simulink model "Kal_noPitch_sim"  (R2023b)
settings: Solver=FixedStepAuto  StartTime=0.0  StopTime=50  FixedStep=0.001  RelTol=1e-3
values from neighbouring files (symbols this model uses):
  beta = pi/10    (= 0.314159265359)    [Kal_noPitch_mat.m]
  cov_ic = cov_ic * (1 + 2*rand)    [Kal_noPitch_mat.m]
  des_vel = [0.1, 0, 0, 0]'    [Kal_noPitch_mat.m]
  eta1 = 0.05    [Kal_noPitch_mat.m]
  eta2 = 0.05    [Kal_noPitch_mat.m]
  G = eye(3) * Ts    [Kal_noPitch_mat.m]
  Gamma = -pi/6    (= -0.523598775598)    [Kal_noPitch_mat.m]
  h_ref = 7    [Kal_noPitch_mat.m]
  init_cond = [2; 0; 0]    [Kal_noPitch_mat.m]
  Kd_dep = (p + 2*damp*wn)*mv(3) + dv(3)    [Control_gains_mat.m]
  Ki_dep = p*(wn^2)*mv(3)    [Control_gains_mat.m]
  Ki_surge = wn^2 * mv(1)    [Control_gains_mat.m]
  Kp_dep = mv(3)*((wn^2) + 2*damp*p*wn)    [Control_gains_mat.m]
  Kp_surge = 2*damp*wn*mv(1) - dv(1)    [Control_gains_mat.m]
  Kt_dep = 1 / sqrt(ti_dep*td_dep)    [Control_gains_mat.m]
  Kt_surge = 1 / ti_surge    [Control_gains_mat.m]
  Lambda = pi/6    (= 0.523598775598)    [Kal_noPitch_mat.m]
  pr0 = [0,0]'    [Kal_noPitch_mat.m]
  Q = zeros(3,3)    [Kal_noPitch_mat.m]
  qt = - 10    (= -10)    [Kal_noPitch_mat.m]
  R = [(eta1^2), 0 ... (first row only)    [Kal_noPitch_mat.m]
  sat_dep = 15    [Model3D_equation_mat.m]
  sat_surge = 15    [Model3D_equation_mat.m]
  sat_tr = 2000    [Model3D_equation_mat.m]
  sig1 = 0.1    [Kal_noPitch_mat.m]
  sig2 = 0.2    [Kal_noPitch_mat.m]
  sig3 = 0.15    [Kal_noPitch_mat.m]
  speed0 = [0.1, 0, 0, 0]'    [Model3D_equation_mat.m]
  Ts = 0.001    [Kal_noPitch_mat.m]
settings Model: Creator=fabio  LastModifiedBy=fabio

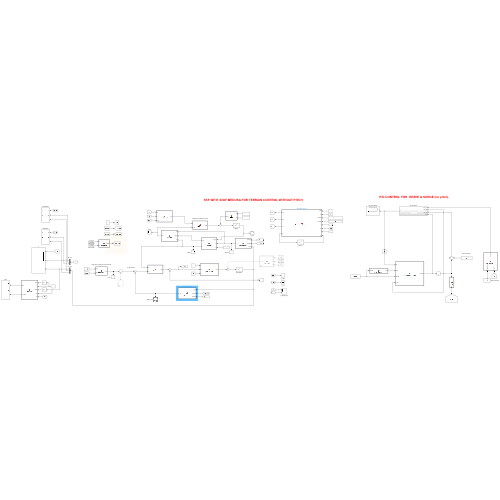
[thumbnail: Simulink's stored preview of the top-level diagram]
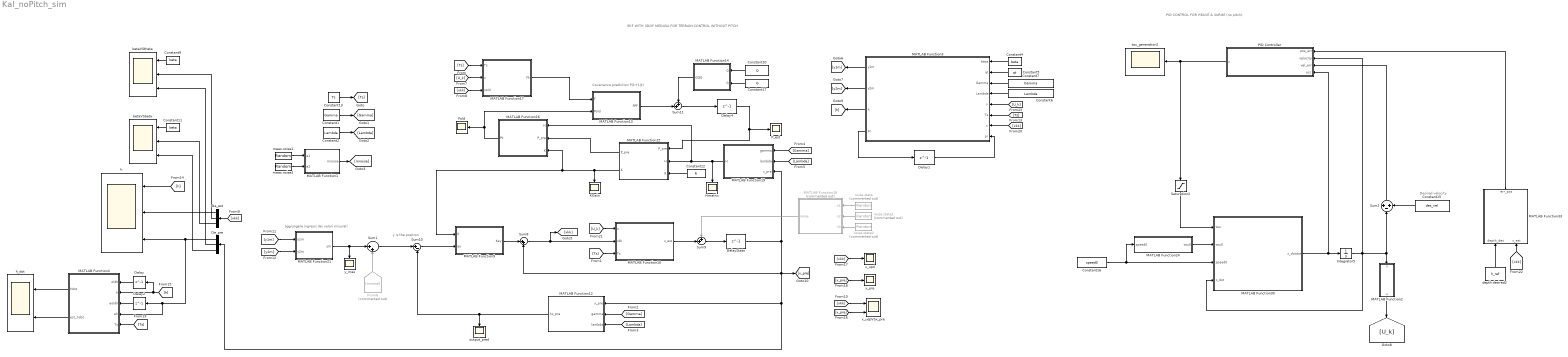
== system Kal_noPitch_sim ==
  note: aggiungere ingressi dei valorì misurati
  note: Covariance prediction P(k+1|k)
  note: EKF WITH 3DOF MEDUSA FOR TERRAIN CONTROL WITHOUT PITCH
  note: y is the position
  note: PID CONTROL FOR HEAVE & SURGE (no pitch).
  note: Desired velocity
  Constant1 : Constant  Value=Gamma
  Constant10 : Constant  Value=Q  VectorParams1D=off
  Constant11 : Constant  Value=beta
  Constant12 : Constant  Value=R
  Constant13 : Constant  Value=Ts
  Constant15 : Constant  Value=des_vel
  Constant16 : Constant  Value=speed0
  Constant17 : Constant  Value=G  VectorParams1D=off
  Constant2 : Constant  Value=Lambda
  Constant4 : Constant  Value=beta
  Constant5 : Constant  Value=qt
  Constant6 : Constant  Value=Lambda
  Constant7 : Constant  Value=Gamma
  Constant9 : Constant  Value=beta
  De_est : Demux  Outputs=3
  De_pre : Demux  Outputs=3
  Delay : Delay  DelayLength=1
  Delay1 : Delay  DelayLength=1  InitialCondition=pr0  UseCircularBuffer=on
  Delay2 : Delay  DelayLength=1
  Delay4 : Delay  DelayLength=1  InitialCondition=cov_ic  UseCircularBuffer=on
  DelayStato : Delay  DelayLength=1  InitialCondition=init_cond  UseCircularBuffer=on
  From6 : From  Commented=on  GotoTag=mnoise
  Hmatrix : Scope
  Integrator5 : Integrator
  KGain : Scope
  MATLAB Function1 : MATLAB Function  TreatAsAtomicUnit=on
  MATLAB Function10 : MATLAB Function  TreatAsAtomicUnit=on
  MATLAB Function12 : MATLAB Function  TreatAsAtomicUnit=on
  MATLAB Function13 : MATLAB Function  TreatAsAtomicUnit=on
  MATLAB Function14 : MATLAB Function  TreatAsAtomicUnit=on
  MATLAB Function15 : MATLAB Function  TreatAsAtomicUnit=on
  MATLAB Function16 : MATLAB Function  TreatAsAtomicUnit=on
  MATLAB Function17 : MATLAB Function  TreatAsAtomicUnit=on
  MATLAB Function18 : MATLAB Function  Commented=on  TreatAsAtomicUnit=on
  MATLAB Function19 : MATLAB Function  TreatAsAtomicUnit=on
  MATLAB Function2 : MATLAB Function  TreatAsAtomicUnit=on
  MATLAB Function21 : MATLAB Function  TreatAsAtomicUnit=on
  MATLAB Function24 : MATLAB Function  TreatAsAtomicUnit=on
  MATLAB Function3 : MATLAB Function  TreatAsAtomicUnit=on
  MATLAB Function30 : MATLAB Function  TreatAsAtomicUnit=on
  MATLAB Function33 : MATLAB Function  TreatAsAtomicUnit=on
  MATLAB Function4 : MATLAB Function  TreatAsAtomicUnit=on
  MATLAB Function9 : MATLAB Function  TreatAsAtomicUnit=on
  PID Controller : Subsystem
  P_est : Scope
  Pold : Scope
  Saturation2 : Saturate  UpperLimit=sat_tr  LowerLimit=-sat_tr
  Sum1 : Sum  Inputs=|++
  Sum10 : Sum  Inputs=|+-
  Sum11 : Sum  Inputs=++|
  Sum2 : Sum  Inputs=+-+
  Sum8 : Sum  Inputs=|++
  Sum9 : Sum  Inputs=++|
  betaVSbeta : Scope  NumInputPorts=3
  betaVStheta : Scope  NumInputPorts=3
  depth desired2 : Constant  Value=h_ref
  h : Scope  NumInputPorts=3
  h_dot : Scope  NumInputPorts=2
  meas.noise1 : RandomNumber  Variance=eta1  SampleTime=Ts
  meas.noise2 : RandomNumber  Variance=eta2  SampleTime=Ts
  noise state : RandomNumber  Commented=on  Variance=sig1  SampleTime=Ts
  noise state1 : RandomNumber  Commented=on  Variance=sig2  SampleTime=Ts
  noise state2 : RandomNumber  Commented=on  Variance=sig3  SampleTime=Ts
  output_pred : Scope
  tau_generation2 : Scope
  x_pre : Scope
  x_udpVSx_pre : Scope  NumInputPorts=2
  x_upd : Scope
  y_mes : Scope
  wires:
  MATLAB Function17/1(Fk) -> MATLAB Function13/1(F)
  DelayStato/1 -> Sum8/2, [x_pre], MATLAB Function12/1(x_pre), De_pre/1, MATLAB Function19/3(x_pre)
  Delay4/1 -> P_est/1, MATLAB Function15/1("P_pre ")
  MATLAB Function12/1(hx_pre) -> Sum10/2, output_pred/1
  Sum10/1 -> MATLAB Function9/2(ey)
  MATLAB Function19/1(H) -> Hmatrix/1, MATLAB Function16/1(H), MATLAB Function15/2(H)
  Constant17/1 -> MATLAB Function14/2(G)
  MATLAB Function14/1(GQG) -> Sum11/1
  MATLAB Function13/1(FPF) -> Sum11/2
  Constant10/1 -> MATLAB Function14/1(Q)
  MATLAB Function10/1(x_est) -> Sum9/2
  MATLAB Function16/1(Pk) -> Pold/1, MATLAB Function13/2(Pold)
  Sum9/1 -> DelayStato/1
  Constant12/1 -> MATLAB Function15/3(R)
  MATLAB Function15/2(K) -> KGain/1, MATLAB Function16/3(K), MATLAB Function9/1(K)
  Sum11/1 -> Delay4/1
  Sum8/1 -> [xkk], MATLAB Function10/2(xkk)
  MATLAB Function15/1(P_pre) -> MATLAB Function16/2(P_pre)
  MATLAB Function9/1(Key) -> Sum8/1
  MATLAB Function21/1(ym) -> y_mes/1, Sum1/1
  Constant13/1 -> [Ts]
  [Ts] -> MATLAB Function17/1(Ts)
  [Ts] -> MATLAB Function10/3(Ts)
  Constant1/1 -> [Gamma]
  Constant2/1 -> [Lambda]
  [Gamma] -> MATLAB Function12/2(gamma)
  [Lambda] -> MATLAB Function12/3(lambda)
  [Gamma] -> MATLAB Function19/1(gamma)
  [Lambda] -> MATLAB Function19/2(lambda)
  noise state/1 -> MATLAB Function18/1(n1)
  noise state2/1 -> MATLAB Function18/3(n3)
  noise state1/1 -> MATLAB Function18/2(n2)
  MATLAB Function18/1(noise) -> Sum9/1
  Sum1/1 -> Sum10/1
  meas.noise1/1 -> MATLAB Function1/1(e1)
  meas.noise2/1 -> MATLAB Function1/2(e2)
  MATLAB Function1/1(mnoise) -> [mnoise]
  [U_k] -> MATLAB Function17/2(u)
  [xkk] -> MATLAB Function17/3(xold)
  Delay1/1 -> MATLAB Function3/8("pr ")
  MATLAB Function3/4(pr) -> Delay1/1
  MATLAB Function3/1(y1m) -> [y1m]
  MATLAB Function3/2(y2m) -> [y2m]
  [y1m] -> MATLAB Function21/1(y1m)
  [y2m] -> MATLAB Function21/2(y2m)
  Constant4/1 -> MATLAB Function3/1(beta)
  Constant5/1 -> MATLAB Function3/2(qt)
  Constant6/1 -> MATLAB Function3/4(Lambda)
  [U_k] -> MATLAB Function3/5(v)
  [Ts] -> MATLAB Function3/6(Ts)
  MATLAB Function3/3(h) -> [h]
  [h] -> h/1
  [xkk] -> De_est/1
  De_est/1 -> h/2
  De_pre/1 -> MATLAB Function4/4(eh), Delay2/1, h/3
  Constant9/1 -> betaVStheta/1
  Constant7/1 -> MATLAB Function3/3(Gamma)
  MATLAB Function4/1(hdot) -> h_dot/1
  De_est/2 -> betaVStheta/2
  De_pre/2 -> betaVStheta/3
  De_est/3 -> betaVSbeta/2
  De_pre/3 -> betaVSbeta/3
  Constant11/1 -> betaVSbeta/1
  [xkk] -> x_udpVSx_pre/1
  [x_pre] -> x_udpVSx_pre/2
  [xkk] -> x_upd/1
  [x_pre] -> x_pre/1
  MATLAB Function4/2(est_hdot) -> h_dot/2
  [h] -> Delay/1, MATLAB Function4/2(h)
  Delay/1 -> MATLAB Function4/1(oldh)
  Delay2/1 -> MATLAB Function4/3(eoldh)
  [Ts] -> MATLAB Function4/5(Ts)
  [xkk] -> MATLAB Function3/7(x)
  From6/1 -> Sum1/2
  Integrator5/1 -> PID Controller/2(velocity), MATLAB Function30/4(x_dot), Sum2/2, MATLAB Function2/1(x)
  MATLAB Function24/1(tau0) -> MATLAB Function30/2(tau0)
  Constant16/1 -> MATLAB Function30/3(speed0), MATLAB Function24/1(speed0)
  Sum2/1 -> PID Controller/3(vel_err)
  PID Controller/1(u) -> tau_generation2/1, Saturation2/1
  MATLAB Function33/1(err_pos) -> PID Controller/1(pos_err)
  MATLAB Function30/1(x_dotdot) -> Integrator5/1, PID Controller/4(acc)
  Saturation2/1 -> MATLAB Function30/1(tau)
  depth desired2/1 -> MATLAB Function33/1(depth_des)
  Constant15/1 -> Sum2/3
  [U_k] -> MATLAB Function10/1(u)
  MATLAB Function2/1(u) -> [U_k]
  [xkk] -> MATLAB Function33/2(x_est)

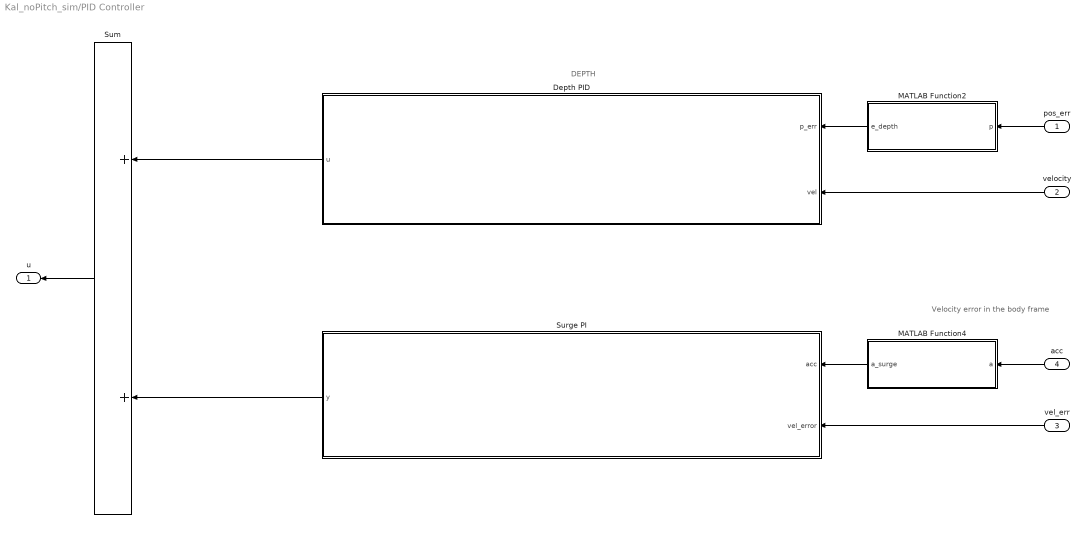
== system Kal_noPitch_sim/PID Controller ==
  note: Velocity error in the body frame
  note: DEPTH
  pos_err : Inport
  velocity : Inport  Port=2
  vel_err : Inport  Port=3
  acc : Inport  Port=4
  Depth PID : Subsystem
  MATLAB Function2 : MATLAB Function  TreatAsAtomicUnit=on
  MATLAB Function4 : MATLAB Function  TreatAsAtomicUnit=on
  Sum : Sum
  Surge PI : Subsystem
  u : Outport
  wires:
  velocity/1 -> Depth PID/2(vel)
  vel_err/1 -> Surge PI/2(vel_error)
  MATLAB Function4/1(a_surge) -> Surge PI/1(acc)
  acc/1 -> MATLAB Function4/1(a)
  Surge PI/1(y) -> Sum/2
  Sum/1 -> u/1
  Depth PID/1(u) -> Sum/1
  pos_err/1 -> MATLAB Function2/1(p)
  MATLAB Function2/1(e_depth) -> Depth PID/1(p_err)

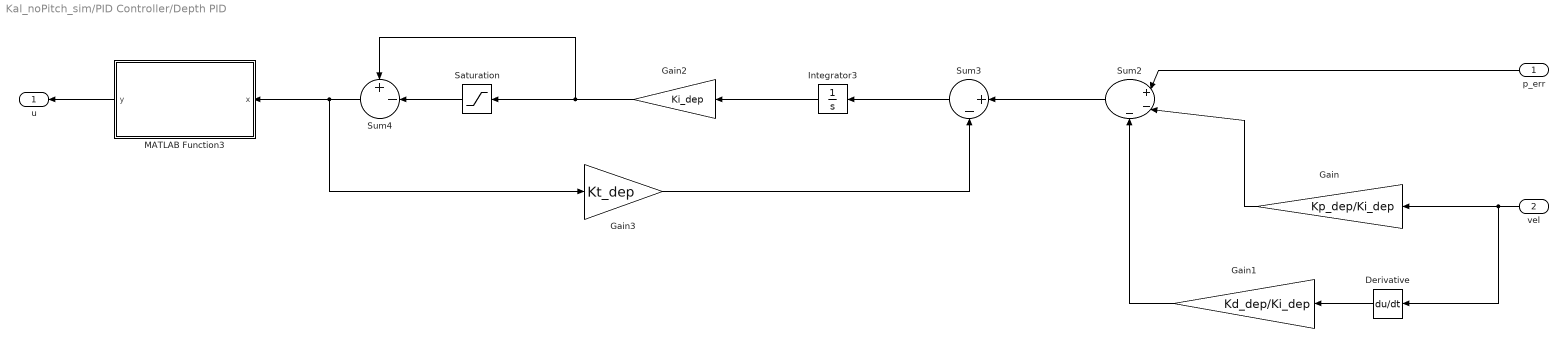
== system Kal_noPitch_sim/PID Controller/Depth PID ==
  p_err : Inport
  vel : Inport  Port=2
  Derivative : Derivative
  Gain : Gain  Gain=Kp_dep/Ki_dep
  Gain1 : Gain  Gain=Kd_dep/Ki_dep
  Gain2 : Gain  Gain=Ki_dep
  Gain3 : Gain  Gain=Kt_dep
  Integrator3 : Integrator
  MATLAB Function3 : MATLAB Function  TreatAsAtomicUnit=on
  Saturation : Saturate  UpperLimit=sat_dep  LowerLimit=-sat_dep
  Sum2 : Sum  Inputs=|+--
  Sum3 : Sum  Inputs=|+-
  Sum4 : Sum  Inputs=+-|
  u : Outport
  wires:
  Sum3/1 -> Integrator3/1
  Integrator3/1 -> Gain2/1
  Gain2/1 -> Sum4/1, Saturation/1
  Sum4/1 -> MATLAB Function3/1(x), Gain3/1
  Derivative/1 -> Gain1/1
  Saturation/1 -> Sum4/2
  Sum2/1 -> Sum3/1
  Gain/1 -> Sum2/2
  Gain1/1 -> Sum2/3
  p_err/1 -> Sum2/1
  vel/1 -> Derivative/1, Gain/1
  MATLAB Function3/1(y) -> u/1
  Gain3/1 -> Sum3/2

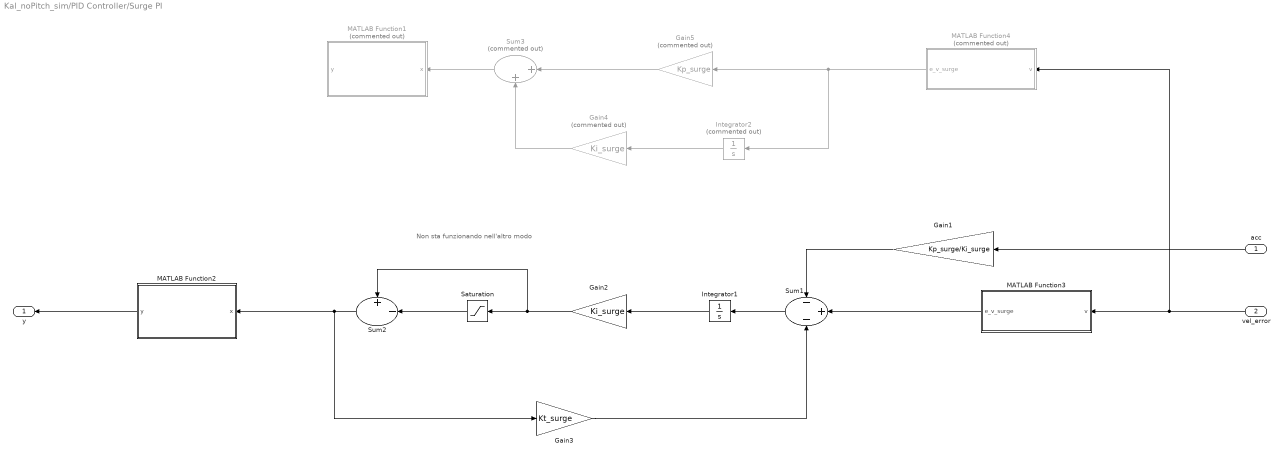
== system Kal_noPitch_sim/PID Controller/Surge PI ==
  note: Non sta funzionando nell'altro modo
  acc : Inport
  vel_error : Inport  Port=2
  Gain1 : Gain  Gain=Kp_surge/Ki_surge
  Gain2 : Gain  Gain=Ki_surge
  Gain3 : Gain  Gain=Kt_surge
  Gain4 : Gain  Commented=on  Gain=Ki_surge
  Gain5 : Gain  Commented=on  Gain=Kp_surge
  Integrator1 : Integrator
  Integrator2 : Integrator  Commented=on
  MATLAB Function1 : MATLAB Function  Commented=on  TreatAsAtomicUnit=on
  MATLAB Function2 : MATLAB Function  TreatAsAtomicUnit=on
  MATLAB Function3 : MATLAB Function  TreatAsAtomicUnit=on
  MATLAB Function4 : MATLAB Function  Commented=on  TreatAsAtomicUnit=on
  Saturation : Saturate  UpperLimit=sat_surge  LowerLimit=-sat_surge
  Sum1 : Sum  Inputs=-+-
  Sum2 : Sum  Inputs=+-|
  Sum3 : Sum  Commented=on  Inputs=|++
  y : Outport
  wires:
  Gain1/1 -> Sum1/1
  Sum2/1 -> Gain3/1, MATLAB Function2/1(x)
  Sum1/1 -> Integrator1/1
  Gain3/1 -> Sum1/3
  Saturation/1 -> Sum2/2
  Gain2/1 -> Sum2/1, Saturation/1
  Integrator1/1 -> Gain2/1
  MATLAB Function3/1(e_v_surge) -> Sum1/2
  Integrator2/1 -> Gain4/1
  vel_error/1 -> MATLAB Function3/1(v), MATLAB Function4/1(v)
  Gain5/1 -> Sum3/1
  Gain4/1 -> Sum3/2
  Sum3/1 -> MATLAB Function1/1(x)
  MATLAB Function4/1(e_v_surge) -> Integrator2/1, Gain5/1
  acc/1 -> Gain1/1
  MATLAB Function2/1(y) -> y/1

== matlab function Kal_noPitch_sim/MATLAB Function14 ==
  data: Q input; GQG output; G input
function GQG = GmatrixQ(Q, G)
    GQG = G*Q*(G');

== matlab function Kal_noPitch_sim/MATLAB Function15 ==
  data: P_pre output; P_pre input; H input; K output; R input
function [P_pre, K] = KalmanGain(P_pre, H, R)
    K = (P_pre*(H'))*pinv((H*P_pre*(H') + R)); 
    K(2,:) = 0; % non sto ancora curando theta

== matlab function Kal_noPitch_sim/MATLAB Function16 ==
  data: H input; P_pre input; Pk output; K input
function Pk = PkComp(H ,P_pre, K)
    s = size((K*H), 1);
    I = eye(s); 
    Pk = (I - K*H)*P_pre;

== matlab function Kal_noPitch_sim/MATLAB Function9 ==
  data: K input; ey input; Key output
function Key = GainMult(K, ey)
    Key = K*ey;

== matlab function Kal_noPitch_sim/MATLAB Function17 ==
  data: Fk output; Ts input; u input; xold input
function Fk = DynamicJacobian(Ts, u, xold)
    delta = xold(3) - xold(2);
    % u(1) = vsurge, u(2) = vheave
    % !! ATTENZIONE:
    % STO CONSIDERANDO H RISPETTO TERRAIN FRAME E THETA E BETA RISPETTO
    % INERZIALE
    F = [0, -u(1)*cos(delta)+u(2)*sin(delta), u(1)*cos(delta)-u(2)*sin(delta);
            0, 0, 0;
            0, 0, 0];
    Fk = eye(3) + Ts * F;

== matlab function Kal_noPitch_sim/MATLAB Function18 ==
  data: n1 input; n2 input; noise output; n3 input
function noise = StateNoise (n1, n2, n3)
    noise = [n1, n2, n3]';

== matlab function Kal_noPitch_sim/MATLAB Function19 ==
  data: gamma input; lambda input; x_pre input; H output
function H = HComputation(gamma, lambda, x_pre)
    % x(1) = h, x(2) = theta, x(3) = beta
    % !! ATTENZIONE:
    % VA MODIFICATO E MESSO CON VALORE ASSOLUTO??
    delta = [(gamma - (x_pre(3) - x_pre(2)));
             (lambda - (x_pre(3) - x_pre(2)))];

    val1 = ((x_pre(1)*sin(delta(1))) / ((cos(delta(1)))^2));
    val2 = ((x_pre(1)*sin(delta(2))) / ((cos(delta(2)))^2)) * sign(cos(delta(1)));

    H = [(1/abs(cos(delta(1)))), val1 * sign(cos(delta(1))), -val1 * sign(cos(delta(1)));
         (1/abs(cos(delta(2)))), val2 * sign(cos(delta(2))), -val2 * sign(cos(delta(2)))];

== matlab function Kal_noPitch_sim/MATLAB Function21 ==
  data: y1m input; y2m input; ym output
function ym = Ymeasured(y1m, y2m) 
    ym = [y1m; y2m];

== matlab function Kal_noPitch_sim/MATLAB Function30 ==
  data: tau input; tau0 input; speed0 input; x_dot input; x_dotdot output
function x_dotdot = vehicle_dynamics_matrix(tau, tau0, speed0, x_dot)
    % updated to medusa model
    m = 30;
    I = 4.14;

    % [surge, sway, heave, roll, pitch, yaw]
    % Added mass
    tau_a = [-25; -2.325; -19.4311; -8.690]; % kl_dot
    
    % Restoring forces
    tau_r = [-0.2; -55.117; 33.6804; -4.14]; % kl
    
    % Hydrodynamic forces
    tau_d = [-19.5; -147.9; -89.4105; -6.23]; % kl_modl
    
    % Virtual mass
    mv = [m; m; m; I] - tau_a;

    % Dissatipative forces
    dv = -tau_r - 2*tau_d .* abs(speed0);

    delta = x_dot - speed0;

    % Accelerations
    % 3 DOF MODEL Linearized
    x_dotdot = zeros(4,1);
    tau(2) = 0;
    
    % surge
    x_dotdot(1) = (tau(1) - tau0(1) - dv(1)*delta(1)) / mv(1); % + mv(2)*speed0(2)*delta(4) + mv(2)*speed0(4)*delta(2)
    % sway
    % x_dotdot(2) = (tau(2) - tau0(2) - dv(2)*delta(2)) / mv(2); % - mv(1)*speed0(1)*delta(4) - mv(1)*speed0(4)*delta(1)
    % heavy
    x_dotdot(3) = (tau(3) - tau0(3) + dv(3)*delta(3)) / mv(3);
    % yaw
    x_dotdot(4) = (tau(4) - tau0(4) - dv(4)*delta(4)) / mv(4); % + (mv(1) - mv(2))*speed0(1)*delta(2) + (mv(1) - mv(2))*speed0(2)*delta(1)
end

== matlab function Kal_noPitch_sim/MATLAB Function1 ==
  data: e1 input; e2 input; mnoise output
function mnoise = StateNoise (e1, e2)
    mnoise = [e1, e2]';

== matlab function Kal_noPitch_sim/MATLAB Function33 ==
  data: depth_des input; x_est input; err_pos output
function err_pos = ErrorComputation(depth_des, x_est)
    h_est = x_est(1);
    err_pos = depth_des - h_est;
    % err_pos(5) = beta - pitch;
end

== matlab function Kal_noPitch_sim/PID Controller/Depth PID/MATLAB Function3 ==
  data: x input; y output
function y = Cond(x)
    y = zeros(4,1);
    y(3) = x(3);
end

== matlab function Kal_noPitch_sim/PID Controller/MATLAB Function4 ==
  data: a_surge output; a input
function a_surge  = Deviator(a)
    a_surge = a(1);
end

== matlab function Kal_noPitch_sim/PID Controller/Surge PI/MATLAB Function1 ==
  data: x input; y output
function y = Cond(x)
    y = zeros(4,1);
    y(1) = x;
end

== matlab function Kal_noPitch_sim/PID Controller/Surge PI/MATLAB Function2 ==
  data: x input; y output
function y = Cond(x)
    y = zeros(4,1);
    y(1) = x;
end

== matlab function Kal_noPitch_sim/PID Controller/Surge PI/MATLAB Function3 ==
  data: e_v_surge output; v input
function e_v_surge  = Deviator(v)
    e_v_surge = v(1);
end

== matlab function Kal_noPitch_sim/PID Controller/Surge PI/MATLAB Function4 ==
  data: e_v_surge output; v input
function e_v_surge  = Deviator(v)
    e_v_surge = v(1);
end

== matlab function Kal_noPitch_sim/MATLAB Function2 ==
  data: x input; u output
function u = temp(x)
    u = zeros (2,1);
    u(1) = x(1);
    u(2) = x(3);
end

== matlab function Kal_noPitch_sim/MATLAB Function3 ==
  data: beta input; qt input; y1m output; Gamma input; Lambda input; v input; Ts input; x input; y2m output; h output; pr input; pr output
function [y1m, y2m, h, pr] = MeasuramentComputation(beta, qt, Gamma, Lambda, v, Ts, x, pr) 
    % terrain construction
    mt = tan(beta);
    m1_g = tan((3*pi/2 + Gamma + x(2)));  
    m2_l = tan((3*pi/2 + Lambda + x(2)));
    % robot position
    % pr(2) = 0 constant 
    pr(1) = pr(1) + Ts * v(1);
    pr(2) = pr(2) - Ts * v(2);
    q1 = pr(2) - m1_g*pr(1);
    q2 = pr(2) - m2_l*pr(1);

    % computation for y1
    xc1 = (q1 - qt) / (mt - m1_g);
    yc1 = mt * xc1 + qt;
    y1m = norm([pr(1) - xc1; pr(2) - yc1]);

    % Computation for y2
    xc2 = (q2 - qt) / (mt - m2_l);
    yc2 = mt * xc2 + qt;
    y2m = norm([pr(1) - xc2; pr(2) - yc2]);
    
    % valore da ottenere di h
    h = (abs(mt*pr(1) - pr(2) + qt))/ (sqrt(mt^2 + 1));
end

== matlab function Kal_noPitch_sim/MATLAB Function4 ==
  data: oldh input; h input; hdot output; eoldh input; eh input; Ts input; est_hdot output
function [hdot, est_hdot] =  Derivation(oldh, h, eoldh, eh, Ts)
    hdot = (h - oldh) / Ts;
    est_hdot = (eh - eoldh) / Ts;

== matlab function Kal_noPitch_sim/MATLAB Function24 ==
  data: tau0 output; speed0 input
function tau0 = tau0Computation(speed0)
    % updated to medusa model
    m = 30;
    I = 4.14;
    g = 9.81;
    WB = -0.8339; % Buoyancy

    % [surge, sway, heave, roll, pitch, yaw]
    % Added mass
    tau_a = [-25; -2.325; -19.4311; -8.690]; % kl_dot
    
    % Restoring forces
    tau_r = [-0.2; -55.117; 33.6804; -4.14]; % kl
    
    % Hydrodynamic forces
    tau_d = [-19.5; -147.9; -89.4105; -6.23]; % kl_modl
    
    % Virtual mass
    mv = [m; m; m; I] - tau_a;

    % Dissatipative forces
    dv = -tau_r - 2*tau_d .* abs(speed0);
    
    % tau0 computation
    tau0 = zeros(4,1);
    tau0(1) = dv(1)*speed0(1); % - mv(2)*speed0(2)*speed0(4)
    tau0(2) = 0; % can do also the equations
    tau0(3) = -dv(3)*speed0(3) - WB;
    % yaw
    tau0(4) = dv(4)*speed0(4); % - (mv(1) - mv(2))*speed0(1)*speed0(2)
    
end

== matlab function Kal_noPitch_sim/PID Controller/MATLAB Function2 ==
  data: p input; e_depth output
function e_depth  = Transformation(p)
    e_depth = - p;
end

== matlab function Kal_noPitch_sim/MATLAB Function10 ==
  data: u input; xkk input; x_est output; Ts input
function x_est = StatePrediction(u, xkk, Ts)
    % xkk(3) = beta, xkk(2) = theta
    % u(1) = vsurge, u(2) = vheave
    A = eye(3);
    delta = xkk(3) - xkk(2);
    B = [-sin(delta), -cos(delta);
         0, 0;
         0, 0];
    x_est = A*xkk + B*u*Ts;

== matlab function Kal_noPitch_sim/MATLAB Function12 ==
  data: x_pre input; hx_pre output; gamma input; lambda input
function hx_pre = OutputPrediction(x_pre, gamma, lambda)
    delta = [(gamma - (x_pre(3) - x_pre(2)));
             (lambda - (x_pre(3) - x_pre(2)))];
    
    hx_pre = [x_pre(1)/abs((cos(delta(1))));
              x_pre(1)/abs((cos(delta(2))))];

== matlab function Kal_noPitch_sim/MATLAB Function13 ==
  data: F input; Pold input; FPF output
function FPF = FPFmatrix(F ,Pold)
    FPF = F*Pold*(F');
